simulink model "CDHRM_model_v1"  (R2019b)
settings: Solver=VariableStepAuto  StartTime=0.0  StopTime=10.0  RelTol=1e-3
InitFcn:
  | parameters.m
values from neighbouring files (symbols this model uses):
  a = 140/1000    (= 0.14)    [parameters.m]
  d = 23/2000    (= 0.0115)    [parameters.m]
  eta = 0.39    [parameters.m]
  g = 9.81    [parameters.m]
  J_L = 0.014 * 10e-7    (= 1.4e-08)    [parameters.m]
  J_R = 0.864 * 10e-7    (= 8.64e-07)    [parameters.m]
  k_m = 2560*100*pi/3    (= 268082.573106)    [parameters.m]
  k_trans = 0.36    [parameters.m]
  l_link = a-2*d    (= 0.117)    [parameters.m]
  m = 0.2    [parameters.m]
  mu_cable = 0.17    [parameters.m]
  n_0 = 9620*pi/30    (= 1007.40404425)    [parameters.m]
  p = 8/1000    (= 0.008)    [parameters.m]
  r = 20.5/1000    (= 0.0205)    [parameters.m]
  r_drum = 0.042    [parameters.m]
undefined symbols (not defined in the file or in its folder): d_drum
libraries: dspindex x18, dspinverses x1, simulink x1
(part 1 of 5)
settings Model: Creator=arund  LastModifiedBy=arund

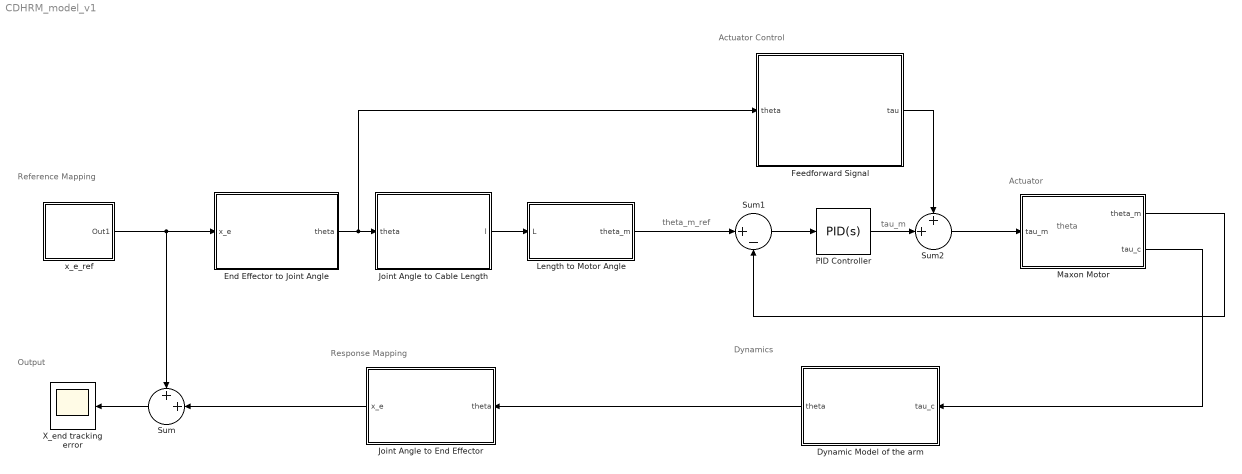
== system CDHRM_model_v1 ==
  note: Actuator
  note: theta_m_ref
  note: Dynamics
  note: Actuator Control
  note: Response Mapping
  note: Output
  note: Reference Mapping
  note: tau_m
  note: theta
  Dynamic Model of the arm : Subsystem
  End Effector to Joint Angle : Subsystem
  Feedforward Signal : Subsystem
  Joint Angle to Cable Length : Subsystem
  Joint Angle to End Effector : Subsystem
  Length to Motor Angle : Subsystem
  Maxon Motor : Subsystem
  PID Controller : simulink/Continuous/PID Controller  Controller=PID  Form=Parallel  TimeDomain=Continuous-time  SampleTime=-1  IntegratorMethod=Forward Euler  FilterMethod=Forward Euler  ControllerParametersSource=internal  P=74.7116129123462  I=0  D=0.141885827214998  UseFilter=on  N=364.6824066771  TunerSelectOption=Transfer Function Based (PID Tuner App)  InitialConditionSource=internal  InitialConditionForIntegrator=0  InitialConditionForFilter=0  DifferentiatorICPrevScaledInput=0  ExternalReset=none  TrackingMode=off  Kt=1  LimitOutput=off  UpperSaturationLimit=inf  LowerSaturationLimit=-inf  LinearizeAsGain=on  AntiWindupMode=none  Kb=1  POutMin=[]  POutMax=[]  IOutMin=[]  IOutMax=[]  DOutMin=[]  DOutMax=[]  NOutMin=[]  NOutMax=[]  SumOutMin=[]  SumOutMax=[]  SaturationOutMin=[]  SaturationOutMax=[]  PParamMin=[]  PParamMax=[]  IParamMin=[]  IParamMax=[]  DParamMin=[]  DParamMax=[]  NParamMin=[]  NParamMax=[]  KbParamMin=[]  KbParamMax=[]  KtParamMin=[]  KtParamMax=[]  KbOutMin=[]  KbOutMax=[]  KtOutMin=[]  KtOutMax=[]  IntegratorOutMin=[]  IntegratorOutMax=[]  FilterOutMin=[]  FilterOutMax=[]  SumI1OutMin=[]  SumI1OutMax=[]  SumI2OutMin=[]  SumI2OutMax=[]  SumI3OutMin=[]  SumI3OutMax=[]  SumI4OutMin=[]  SumI4OutMax=[]  SumDOutMin=[]  SumDOutMax=[]  DifferentiatorOutMin=[]  DifferentiatorOutMax=[]  FilterDiffOutCoefMin=[]  FilterDiffOutCoefMax=[]  ReciprocalOutMin=[]  ReciprocalOutMax=[]  SumDenOutMin=[]  SumDenOutMax=[]  SumNumOutMin=[]  SumNumOutMax=[]  DivideOutMin=[]  DivideOutMax=[]  IntegratorContinuousStateAttributes=''  IntegratorStateMustResolveToSignalObject=off  IntegratorRTWStateStorageClass=Auto  FilterContinuousStateAttributes=''  FilterStateMustResolveToSignalObject=off  FilterRTWStateStorageClass=Auto  ParallelPVariant=InternalParameters  IdealPVariant=Disabled  IVariant=InternalParameters  DVariant=InternalParameters  IntegratorVariant=Continuous  SatVariant=Disabled  AWVariant=Passthrough  PCopyVariant=Disabled  TRVariant=Disabled  FdbkBlocksVariant=Forward  IdealPFdbkVariant=Disabled  SatFdbkVariant=Disabled  DerivativeFilterVariant=ContFilter  NVariant=InternalParameters  NCopyVariant=Disabled  FilterICVariant=InternalICsFilter  IntegratorICVariant=InternalICs  ExternalResetVariant=Disabled  TRSumVariant=Passthrough  SumFdbkVariant=Disabled  SumVariant=Sum_PID
  Sum : Sum  Inputs=++|
  Sum1 : Sum  Inputs=|+-
  Sum2 : Sum  Inputs=++|
  X_end tracking error : Scope
  x_e_ref : Subsystem
  wires:
  Sum/1 -> X_end tracking error/1
  Joint Angle to End Effector/1(x_e) -> Sum/2
  Length to Motor Angle/1(theta_m) -> Sum1/1
  Sum1/1 -> PID Controller/1
  Maxon Motor/1(theta_m) -> Sum1/2
  Joint Angle to Cable Length/1(l) -> Length to Motor Angle/1(L)
  Sum2/1 -> Maxon Motor/1(tau_m)
  Dynamic Model of the arm/1(theta) -> Joint Angle to End Effector/1(theta)
  PID Controller/1 -> Sum2/2
  x_e_ref/1(Out1) -> End Effector to Joint Angle/1(x_e), Sum/1
  Maxon Motor/2(tau_c) -> Dynamic Model of the arm/1(tau_c)
  Feedforward Signal/1(tau) -> Sum2/1
  End Effector to Joint Angle/1(theta) -> Feedforward Signal/1(theta), Joint Angle to Cable Length/1(theta)

== system CDHRM_model_v1/Dynamic Model of the arm ==
  tau_c : Inport
  Integrator : Integrator
  Integrator1 : Integrator
  M_inv(theta) : Subsystem
  Matrix Multiply : Product  Multiplication=Matrix(*)
  h(theta,d_theta) : Subsystem
  theta : Outport
  wires:
  Integrator/1 -> h(theta,d_theta)/2(d_theta), Integrator1/1  "d_theta"
  Integrator1/1 -> h(theta,d_theta)/1(theta), M_inv(theta)/1(theta), theta/1
  Matrix Multiply/1 -> Integrator/1  "dd_theta"
  M_inv(theta)/1(M_inv) -> Matrix Multiply/1
  tau_c/1 -> M_inv(theta)/2(tau_c), h(theta,d_theta)/3(tau_c)
  h(theta,d_theta)/1(h) -> Matrix Multiply/2

== system CDHRM_model_v1/End Effector to Joint Angle ==
  x_e : Inport
  Constant1 : Constant  Value=a
  "End Effector to Joint Angle " : MATLAB Function  TreatAsAtomicUnit=on
  Memory : Memory
  Memory1 : Memory
  theta : Outport
  wires:
  "End Effector to Joint Angle "/1(theta) -> theta/1, Memory1/1
  Memory1/1 -> "End Effector to Joint Angle "/4(theta_prev)
  Memory/1 -> "End Effector to Joint Angle "/3(x_e_prev)
  x_e/1 -> Memory/1, "End Effector to Joint Angle "/2(x_e)
  Constant1/1 -> "End Effector to Joint Angle "/1(a)

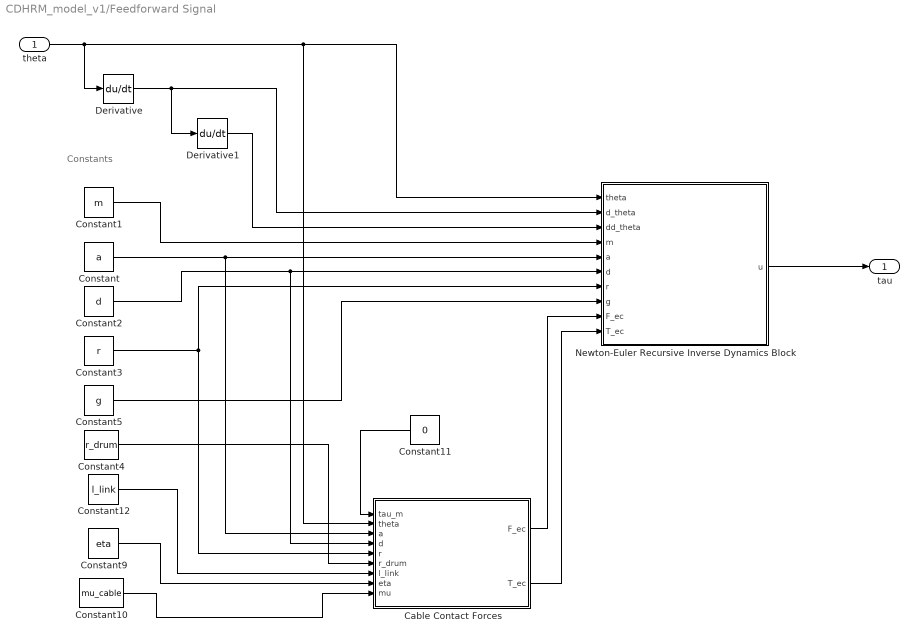
== system CDHRM_model_v1/Feedforward Signal ==
  note: Constants
  theta : Inport
  Cable Contact Forces : MATLAB Function  TreatAsAtomicUnit=on
  Constant : Constant  Value=a
  Constant1 : Constant  Value=m
  Constant10 : Constant  Value=mu_cable
  Constant11 : Constant  Value=0
  Constant12 : Constant  Value=l_link
  Constant2 : Constant  Value=d
  Constant3 : Constant  Value=r
  Constant4 : Constant  Value=r_drum
  Constant5 : Constant  Value=g
  Constant9 : Constant  Value=eta
  Derivative : Derivative  CoefficientInTFapproximation=0
  Derivative1 : Derivative  CoefficientInTFapproximation=0
  Newton-Euler Recursive Inverse Dynamics Block : MATLAB Function  TreatAsAtomicUnit=on
  tau : Outport
  wires:
  Constant/1 -> Cable Contact Forces/3(a), Newton-Euler Recursive Inverse Dynamics Block/5(a)
  Constant9/1 -> Cable Contact Forces/8(eta)
  Constant4/1 -> Cable Contact Forces/6(r_drum)
  theta/1 -> Derivative/1, Cable Contact Forces/2(theta), Newton-Euler Recursive Inverse Dynamics Block/1(theta)
  Constant2/1 -> Cable Contact Forces/4(d), Newton-Euler Recursive Inverse Dynamics Block/6(d)
  Constant3/1 -> Cable Contact Forces/5(r), Newton-Euler Recursive Inverse Dynamics Block/7(r)
  Constant10/1 -> Cable Contact Forces/9(mu)
  Constant1/1 -> Newton-Euler Recursive Inverse Dynamics Block/4(m)
  Constant5/1 -> Newton-Euler Recursive Inverse Dynamics Block/8(g)
  Newton-Euler Recursive Inverse Dynamics Block/1(u) -> tau/1
  Cable Contact Forces/2(T_ec) -> Newton-Euler Recursive Inverse Dynamics Block/10(T_ec)
  Cable Contact Forces/1(F_ec) -> Newton-Euler Recursive Inverse Dynamics Block/9(F_ec)
  Constant12/1 -> Cable Contact Forces/7(l_link)
  Constant11/1 -> Cable Contact Forces/1(tau_m)
  Derivative/1 -> Derivative1/1, Newton-Euler Recursive Inverse Dynamics Block/2(d_theta)
  Derivative1/1 -> Newton-Euler Recursive Inverse Dynamics Block/3(dd_theta)

== system CDHRM_model_v1/Joint Angle to Cable Length ==
  theta : Inport
  Joint Angle to Cable Length : MATLAB Function  TreatAsAtomicUnit=on
  theta to phi : MATLAB Function  TreatAsAtomicUnit=on
  l : Outport
  wires:
  Joint Angle to Cable Length/1(l) -> l/1
  theta/1 -> theta to phi/1(theta)
  theta to phi/1(phi_p) -> Joint Angle to Cable Length/1(phi_p)
  theta to phi/2(phi_d) -> Joint Angle to Cable Length/2(phi_d)

== system CDHRM_model_v1/Joint Angle to End Effector ==
  theta : Inport
  Constant1 : Constant  Value=a
  Derivative : Derivative  CoefficientInTFapproximation=0
  Integrator : Integrator
  "Jacobian of theta " : MATLAB Function  TreatAsAtomicUnit=on
  MatrixMultiply : Product  Multiplication=Matrix(*)
  x_e : Outport
  wires:
  Derivative/1 -> MatrixMultiply/2
  "Jacobian of theta "/1(J) -> MatrixMultiply/1
  Constant1/1 -> "Jacobian of theta "/1(a)
  theta/1 -> "Jacobian of theta "/2(theta), Derivative/1
  MatrixMultiply/1 -> Integrator/1
  Integrator/1 -> x_e/1

== system CDHRM_model_v1/Length to Motor Angle ==
  L : Inport
  Constant : Constant  Value=p
  Constant2 : Constant  Value=d_drum
  Divide : Product  Inputs=*/
  Transmission ratio : Subsystem
  theta_m : Outport
  wires:
  L/1 -> Divide/1
  Constant2/1 -> Transmission ratio/2(d_drum)
  Constant/1 -> Transmission ratio/1(p)
  Transmission ratio/1(k) -> Divide/2
  Divide/1 -> theta_m/1

== system CDHRM_model_v1/Maxon Motor ==
  tau_m : Inport
  Motor : Subsystem
  Speed to Torque : Subsystem
  theta_m : Outport
  tau_c : Outport  Port=2
  wires:
  tau_m/1 -> Motor/1(tau_m)
  Motor/1(Out1) -> theta_m/1
  Motor/2(Out2) -> Speed to Torque/1(d_theta_m)
  Speed to Torque/1(tau_c) -> tau_c/1

== system CDHRM_model_v1/x_e_ref ==
  Mux : Mux  Inputs=6
  X_end_ref{,1..4} (5 alike) : Step  After=0  SampleTime=0
  X_end_ref5 : Step  After=0.1  SampleTime=0
  Out1 : Outport
  wires:
  Mux/1 -> Out1/1
  X_end_ref5/1 -> Mux/1
  X_end_ref/1 -> Mux/2
  X_end_ref1/1 -> Mux/3
  X_end_ref2/1 -> Mux/4
  X_end_ref3/1 -> Mux/5
  X_end_ref4/1 -> Mux/6

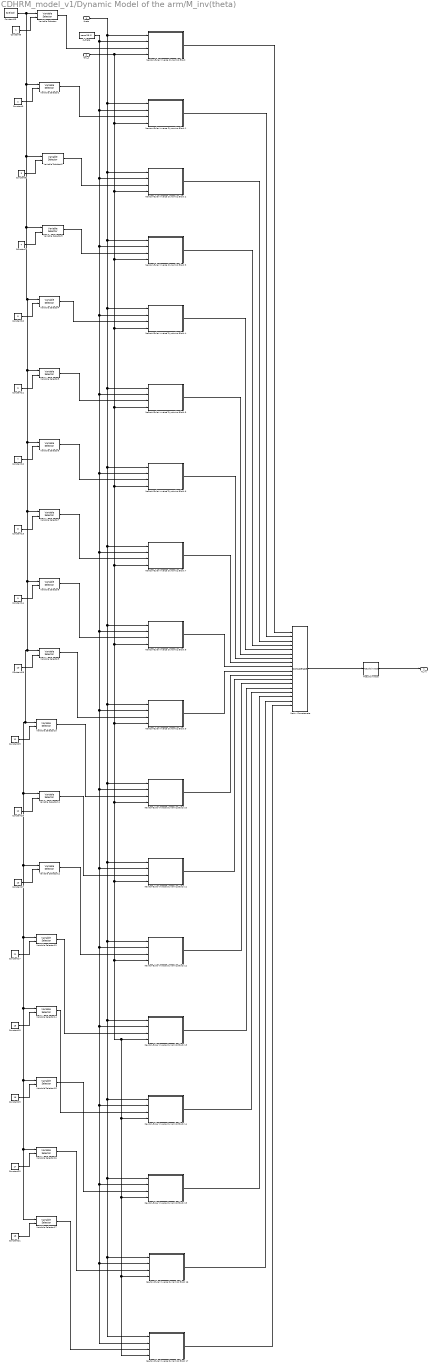
== system CDHRM_model_v1/Dynamic Model of the arm/M_inv(theta) ==
  theta : Inport
  tau_c : Inport  Port=2
  Constant10 : Constant  Value=5
  Constant11 : Constant  Value=6
  Constant12 : Constant  Value=7
  Constant13 : Constant  Value=8
  Constant14 : Constant  Value=9
  Constant15 : Constant  Value=eye(18)
  Constant17 : Constant  Value=14
  Constant18 : Constant  Value=15
  Constant19 : Constant  Value=16
  Constant20 : Constant  Value=17
  Constant21 : Constant  Value=18
  Constant26 : Constant  Value=12
  Constant27 : Constant  Value=13
  Constant28 : Constant  Value=10
  Constant29 : Constant  Value=11
  Constant6 : Constant  Value=3
  Constant7 : Constant  Value=4
  Constant8 : Constant
  Constant9 : Constant  Value=2
  Matrix Concatenate : Concatenate  NumInputs=18  Mode=Multidimensional array  ConcatenateDimension=2
  "Newton-Euler Inverse Dynamics Block " : Subsystem
  Newton-Euler Inverse Dynamics Block 1 : Subsystem
  Newton-Euler Inverse Dynamics Block 10 : Subsystem
  Newton-Euler Inverse Dynamics Block 11 : Subsystem
  Newton-Euler Inverse Dynamics Block 12 : Subsystem
  Newton-Euler Inverse Dynamics Block 13 : Subsystem
  Newton-Euler Inverse Dynamics Block 14 : Subsystem
  Newton-Euler Inverse Dynamics Block 15 : Subsystem
  Newton-Euler Inverse Dynamics Block 16 : Subsystem
  Newton-Euler Inverse Dynamics Block 17 : Subsystem
  Newton-Euler Inverse Dynamics Block 2 : Subsystem
  Newton-Euler Inverse Dynamics Block 3 : Subsystem
  Newton-Euler Inverse Dynamics Block 4 : Subsystem
  Newton-Euler Inverse Dynamics Block 5 : Subsystem
  Newton-Euler Inverse Dynamics Block 6 : Subsystem
  Newton-Euler Inverse Dynamics Block 7 : Subsystem
  Newton-Euler Inverse Dynamics Block 8 : Subsystem
  Newton-Euler Inverse Dynamics Block 9 : Subsystem
  Pseudoinverse : dspinverses/Pseudoinverse  wanterr=off  SimulateUsing=Interpreted execution
      settings: SourceProductName=DSP System Toolbox  SourceProductBaseCode=DS
  Variable Selector{,1..17} (18 alike) : dspindex/Variable Selector  NumInputs=1  rowsOrCols=Columns  IdxMode=Variable  Elements=[1 3]  ZerOneIdxMode=One-based  errmode=Clip Index  FillMode=on  FillValues=0
  d_theta : Constant  Value=zeros(18,1)
  M_inv : Outport
  wires:
  Variable Selector/1 -> "Newton-Euler Inverse Dynamics Block "/3(dd_theta)
  Constant8/1 -> Variable Selector/2
  Variable Selector1/1 -> Newton-Euler Inverse Dynamics Block 1/3(dd_theta)
  Constant9/1 -> Variable Selector1/2
  Matrix Concatenate/1 -> Pseudoinverse/1
  Constant6/1 -> Variable Selector2/2
  Variable Selector2/1 -> Newton-Euler Inverse Dynamics Block 2/3(dd_theta)
  Constant7/1 -> Variable Selector3/2
  Variable Selector3/1 -> Newton-Euler Inverse Dynamics Block 3/3(dd_theta)
  Constant10/1 -> Variable Selector4/2
  Variable Selector4/1 -> Newton-Euler Inverse Dynamics Block 4/3(dd_theta)
  Constant11/1 -> Variable Selector5/2
  Variable Selector5/1 -> Newton-Euler Inverse Dynamics Block 5/3(dd_theta)
  Constant12/1 -> Variable Selector6/2
  Variable Selector6/1 -> Newton-Euler Inverse Dynamics Block 6/3(dd_theta)
  Constant13/1 -> Variable Selector7/2
  Variable Selector7/1 -> Newton-Euler Inverse Dynamics Block 7/3(dd_theta)
  Constant14/1 -> Variable Selector8/2
  Variable Selector8/1 -> Newton-Euler Inverse Dynamics Block 8/3(dd_theta)
  Pseudoinverse/1 -> M_inv/1
  Variable Selector11/1 -> Newton-Euler Inverse Dynamics Block 11/3(dd_theta)
  Constant26/1 -> Variable Selector11/2
  Variable Selector14/1 -> Newton-Euler Inverse Dynamics Block 14/3(dd_theta)
  Constant18/1 -> Variable Selector14/2
  Variable Selector17/1 -> Newton-Euler Inverse Dynamics Block 17/3(dd_theta)
  Constant21/1 -> Variable Selector17/2
  Constant15/1 -> Variable Selector9/1, Variable Selector10/1, Variable Selector17/1, Variable Selector16/1, Variable Selector15/1, Variable Selector14/1, Variable Selector13/1, Variable Selector12/1, Variable Selector11/1, Variable Selector8/1, Variable Selector7/1, Variable Selector6/1, Variable Selector5/1, Variable Selector4/1, Variable Selector3/1, Variable Selector2/1, Variable Selector1/1, Variable Selector/1
  d_theta/1 -> "Newton-Euler Inverse Dynamics Block "/2(d_theta), Newton-Euler Inverse Dynamics Block 6/2(d_theta), Newton-Euler Inverse Dynamics Block 7/2(d_theta), Newton-Euler Inverse Dynamics Block 8/2(d_theta), Newton-Euler Inverse Dynamics Block 9/2(d_theta), Newton-Euler Inverse Dynamics Block 11/2(d_theta), Newton-Euler Inverse Dynamics Block 12/2(d_theta), Newton-Euler Inverse Dynamics Block 17/2(d_theta), Newton-Euler Inverse Dynamics Block 16/2(d_theta), Newton-Euler Inverse Dynamics Block 15/2(d_theta), Newton-Euler Inverse Dynamics Block 14/2(d_theta), Newton-Euler Inverse Dynamics Block 13/2(d_theta), Newton-Euler Inverse Dynamics Block 10/2(d_theta), Newton-Euler Inverse Dynamics Block 5/2(d_theta), Newton-Euler Inverse Dynamics Block 4/2(d_theta), Newton-Euler Inverse Dynamics Block 3/2(d_theta), Newton-Euler Inverse Dynamics Block 2/2(d_theta), Newton-Euler Inverse Dynamics Block 1/2(d_theta)
  theta/1 -> "Newton-Euler Inverse Dynamics Block "/1(theta), Newton-Euler Inverse Dynamics Block 1/1(theta), Newton-Euler Inverse Dynamics Block 3/1(theta), Newton-Euler Inverse Dynamics Block 4/1(theta), Newton-Euler Inverse Dynamics Block 5/1(theta), Newton-Euler Inverse Dynamics Block 6/1(theta), Newton-Euler Inverse Dynamics Block 7/1(theta), Newton-Euler Inverse Dynamics Block 8/1(theta), Newton-Euler Inverse Dynamics Block 9/1(theta), Newton-Euler Inverse Dynamics Block 10/1(theta), Newton-Euler Inverse Dynamics Block 11/1(theta), Newton-Euler Inverse Dynamics Block 12/1(theta), Newton-Euler Inverse Dynamics Block 13/1(theta), Newton-Euler Inverse Dynamics Block 14/1(theta), Newton-Euler Inverse Dynamics Block 16/1(theta), Newton-Euler Inverse Dynamics Block 17/1(theta), Newton-Euler Inverse Dynamics Block 15/1(theta), Newton-Euler Inverse Dynamics Block 2/1(theta)
  Constant28/1 -> Variable Selector9/2
  Variable Selector13/1 -> Newton-Euler Inverse Dynamics Block 13/3(dd_theta)
  Constant17/1 -> Variable Selector13/2
  Constant20/1 -> Variable Selector16/2
  Constant19/1 -> Variable Selector15/2
  Constant29/1 -> Variable Selector10/2
  Variable Selector10/1 -> Newton-Euler Inverse Dynamics Block 10/3(dd_theta)
  Variable Selector9/1 -> Newton-Euler Inverse Dynamics Block 9/3(dd_theta)
  Constant27/1 -> Variable Selector12/2
  Variable Selector12/1 -> Newton-Euler Inverse Dynamics Block 12/3(dd_theta)
  Variable Selector15/1 -> Newton-Euler Inverse Dynamics Block 15/3(dd_theta)
  Variable Selector16/1 -> Newton-Euler Inverse Dynamics Block 16/3(dd_theta)
  tau_c/1 -> Newton-Euler Inverse Dynamics Block 6/4(tau_c), Newton-Euler Inverse Dynamics Block 11/4(tau_c), Newton-Euler Inverse Dynamics Block 12/4(tau_c), Newton-Euler Inverse Dynamics Block 13/4(tau_c), Newton-Euler Inverse Dynamics Block 14/4(tau_c), Newton-Euler Inverse Dynamics Block 15/4(tau_c), Newton-Euler Inverse Dynamics Block 17/4(tau_c), Newton-Euler Inverse Dynamics Block 16/4(tau_c), Newton-Euler Inverse Dynamics Block 10/4(tau_c), Newton-Euler Inverse Dynamics Block 9/4(tau_c), Newton-Euler Inverse Dynamics Block 8/4(tau_c), Newton-Euler Inverse Dynamics Block 7/4(tau_c), Newton-Euler Inverse Dynamics Block 5/4(tau_c), Newton-Euler Inverse Dynamics Block 4/4(tau_c), Newton-Euler Inverse Dynamics Block 3/4(tau_c), Newton-Euler Inverse Dynamics Block 2/4(tau_c), Newton-Euler Inverse Dynamics Block 1/4(tau_c), "Newton-Euler Inverse Dynamics Block "/4(tau_c)
  "Newton-Euler Inverse Dynamics Block "/1(tau) -> Matrix Concatenate/1
  Newton-Euler Inverse Dynamics Block 1/1(tau) -> Matrix Concatenate/2
  Newton-Euler Inverse Dynamics Block 2/1(tau) -> Matrix Concatenate/3
  Newton-Euler Inverse Dynamics Block 3/1(tau) -> Matrix Concatenate/4
  Newton-Euler Inverse Dynamics Block 4/1(tau) -> Matrix Concatenate/5
  Newton-Euler Inverse Dynamics Block 5/1(tau) -> Matrix Concatenate/6
  Newton-Euler Inverse Dynamics Block 6/1(tau) -> Matrix Concatenate/7
  Newton-Euler Inverse Dynamics Block 7/1(tau) -> Matrix Concatenate/8
  Newton-Euler Inverse Dynamics Block 8/1(tau) -> Matrix Concatenate/9
  Newton-Euler Inverse Dynamics Block 9/1(tau) -> Matrix Concatenate/10
  Newton-Euler Inverse Dynamics Block 10/1(tau) -> Matrix Concatenate/11
  Newton-Euler Inverse Dynamics Block 11/1(tau) -> Matrix Concatenate/12
  Newton-Euler Inverse Dynamics Block 12/1(tau) -> Matrix Concatenate/13
  Newton-Euler Inverse Dynamics Block 13/1(tau) -> Matrix Concatenate/14
  Newton-Euler Inverse Dynamics Block 14/1(tau) -> Matrix Concatenate/15
  Newton-Euler Inverse Dynamics Block 15/1(tau) -> Matrix Concatenate/16
  Newton-Euler Inverse Dynamics Block 16/1(tau) -> Matrix Concatenate/17
  Newton-Euler Inverse Dynamics Block 17/1(tau) -> Matrix Concatenate/18

== system CDHRM_model_v1/Dynamic Model of the arm/h(theta,d_theta) ==
  theta : Inport
  d_theta : Inport  Port=2
  tau_c : Inport  Port=3
  "Newton-Euler Inverse Dynamics Block " : Subsystem
  dd_theta : Constant  Value=zeros(18,1)
  h : Outport
  wires:
  "Newton-Euler Inverse Dynamics Block "/1(tau) -> h/1
  dd_theta/1 -> "Newton-Euler Inverse Dynamics Block "/3(dd_theta)
  d_theta/1 -> "Newton-Euler Inverse Dynamics Block "/2(d_theta)
  theta/1 -> "Newton-Euler Inverse Dynamics Block "/1(theta)
  tau_c/1 -> "Newton-Euler Inverse Dynamics Block "/4(tau_c)

== system CDHRM_model_v1/Length to Motor Angle/Transmission ratio ==
  p : Inport
  d_drum : Inport  Port=2
  Multiply : Gain  Gain=k_trans
  Square : Math  Operator=square  SignedPower=off  SaturateOnIntegerOverflow=on
  Square Root : Sqrt  SaturateOnIntegerOverflow=on
  Square1 : Math  Operator=square  SignedPower=off  SaturateOnIntegerOverflow=on
  Sum : Sum
  k : Outport
  wires:
  Square/1 -> Sum/1
  p/1 -> Square/1
  d_drum/1 -> Square1/1
  Square1/1 -> Sum/2
  Sum/1 -> Square Root/1
  Square Root/1 -> Multiply/1
  Multiply/1 -> k/1

== system CDHRM_model_v1/Maxon Motor/Motor ==
  tau_m : Inport
  Add : Sum
  Constant1 : Constant  Value=J_L
  Constant2 : Constant  Value=J_R
  Integrator : Integrator
  Integrator1 : Integrator
  Product : Product  Inputs=*/
  Out1 : Outport
  Out2 : Outport  Port=2
  wires:
  Integrator/1 -> Out1/1
  Integrator1/1 -> Out2/1, Integrator/1
  Product/1 -> Integrator1/1
  Constant2/1 -> Add/2
  tau_m/1 -> Product/1
  Add/1 -> Product/2
  Constant1/1 -> Add/1

== system CDHRM_model_v1/Maxon Motor/Speed to Torque ==
  d_theta_m : Inport
  Constant : Constant  Value=k_m
  Constant1 : Constant  Value=n_0
  Divide : Product  Inputs=*/
  Subtract : Sum  Inputs=+-
  tau_c : Outport
  wires:
  Constant/1 -> Divide/2
  Constant1/1 -> Subtract/1
  Divide/1 -> tau_c/1
  Subtract/1 -> Divide/1
  d_theta_m/1 -> Subtract/2

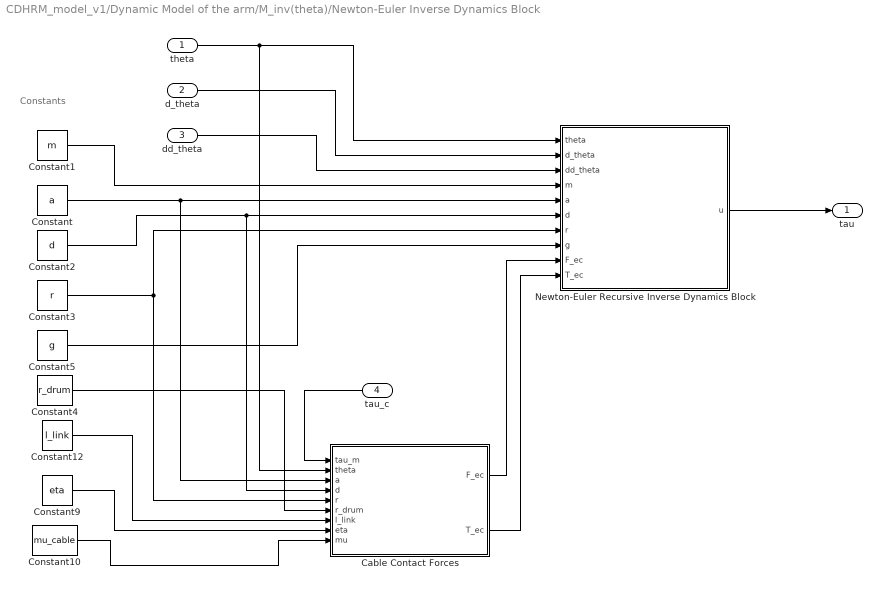
== system CDHRM_model_v1/Dynamic Model of the arm/M_inv(theta)/Newton-Euler Inverse Dynamics Block  ==
  note: Constants
  theta : Inport
  d_theta : Inport  Port=2
  dd_theta : Inport  Port=3
  tau_c : Inport  Port=4
  Cable Contact Forces : MATLAB Function  TreatAsAtomicUnit=on
  Constant : Constant  Value=a
  Constant1 : Constant  Value=m
  Constant10 : Constant  Value=mu_cable
  Constant12 : Constant  Value=l_link
  Constant2 : Constant  Value=d
  Constant3 : Constant  Value=r
  Constant4 : Constant  Value=r_drum
  Constant5 : Constant  Value=g
  Constant9 : Constant  Value=eta
  Newton-Euler Recursive Inverse Dynamics Block : MATLAB Function  TreatAsAtomicUnit=on
  tau : Outport
  wires:
  Constant/1 -> Cable Contact Forces/3(a), Newton-Euler Recursive Inverse Dynamics Block/5(a)
  dd_theta/1 -> Newton-Euler Recursive Inverse Dynamics Block/3(dd_theta)
  Constant9/1 -> Cable Contact Forces/8(eta)
  Constant4/1 -> Cable Contact Forces/6(r_drum)
  theta/1 -> Newton-Euler Recursive Inverse Dynamics Block/1(theta), Cable Contact Forces/2(theta)
  Constant2/1 -> Cable Contact Forces/4(d), Newton-Euler Recursive Inverse Dynamics Block/6(d)
  Constant3/1 -> Cable Contact Forces/5(r), Newton-Euler Recursive Inverse Dynamics Block/7(r)
  Constant10/1 -> Cable Contact Forces/9(mu)
  d_theta/1 -> Newton-Euler Recursive Inverse Dynamics Block/2(d_theta)
  Constant1/1 -> Newton-Euler Recursive Inverse Dynamics Block/4(m)
  Constant5/1 -> Newton-Euler Recursive Inverse Dynamics Block/8(g)
  Newton-Euler Recursive Inverse Dynamics Block/1(u) -> tau/1
  Cable Contact Forces/2(T_ec) -> Newton-Euler Recursive Inverse Dynamics Block/10(T_ec)
  Cable Contact Forces/1(F_ec) -> Newton-Euler Recursive Inverse Dynamics Block/9(F_ec)
  Constant12/1 -> Cable Contact Forces/7(l_link)
  tau_c/1 -> Cable Contact Forces/1(tau_m)

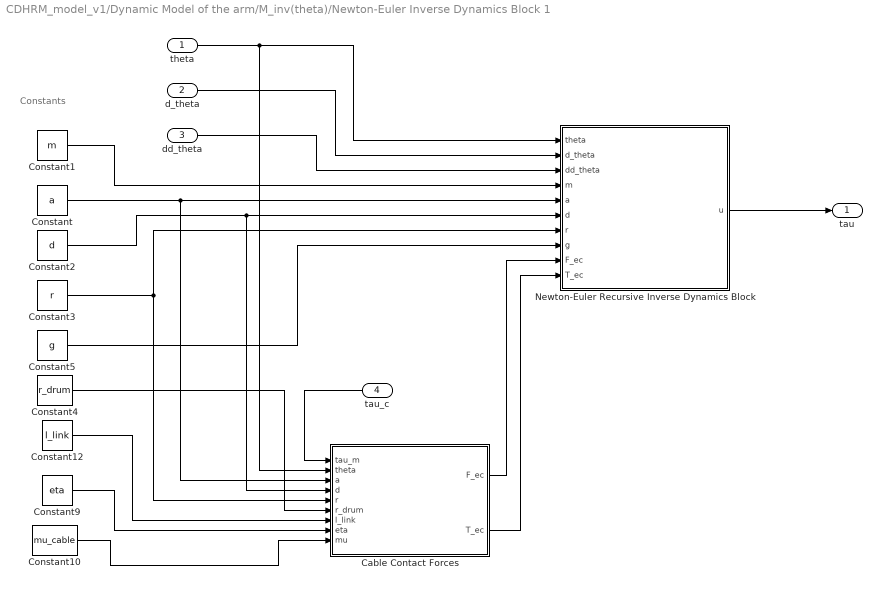
== system CDHRM_model_v1/Dynamic Model of the arm/M_inv(theta)/Newton-Euler Inverse Dynamics Block 1 ==
  note: Constants
  theta : Inport
  d_theta : Inport  Port=2
  dd_theta : Inport  Port=3
  tau_c : Inport  Port=4
  Cable Contact Forces : MATLAB Function  TreatAsAtomicUnit=on
  Constant : Constant  Value=a
  Constant1 : Constant  Value=m
  Constant10 : Constant  Value=mu_cable
  Constant12 : Constant  Value=l_link
  Constant2 : Constant  Value=d
  Constant3 : Constant  Value=r
  Constant4 : Constant  Value=r_drum
  Constant5 : Constant  Value=g
  Constant9 : Constant  Value=eta
  Newton-Euler Recursive Inverse Dynamics Block : MATLAB Function  TreatAsAtomicUnit=on
  tau : Outport
  wires:
  Constant/1 -> Cable Contact Forces/3(a), Newton-Euler Recursive Inverse Dynamics Block/5(a)
  dd_theta/1 -> Newton-Euler Recursive Inverse Dynamics Block/3(dd_theta)
  Constant9/1 -> Cable Contact Forces/8(eta)
  Constant4/1 -> Cable Contact Forces/6(r_drum)
  theta/1 -> Newton-Euler Recursive Inverse Dynamics Block/1(theta), Cable Contact Forces/2(theta)
  Constant2/1 -> Cable Contact Forces/4(d), Newton-Euler Recursive Inverse Dynamics Block/6(d)
  Constant3/1 -> Cable Contact Forces/5(r), Newton-Euler Recursive Inverse Dynamics Block/7(r)
  Constant10/1 -> Cable Contact Forces/9(mu)
  d_theta/1 -> Newton-Euler Recursive Inverse Dynamics Block/2(d_theta)
  Constant1/1 -> Newton-Euler Recursive Inverse Dynamics Block/4(m)
  Constant5/1 -> Newton-Euler Recursive Inverse Dynamics Block/8(g)
  Newton-Euler Recursive Inverse Dynamics Block/1(u) -> tau/1
  Cable Contact Forces/2(T_ec) -> Newton-Euler Recursive Inverse Dynamics Block/10(T_ec)
  Cable Contact Forces/1(F_ec) -> Newton-Euler Recursive Inverse Dynamics Block/9(F_ec)
  Constant12/1 -> Cable Contact Forces/7(l_link)
  tau_c/1 -> Cable Contact Forces/1(tau_m)

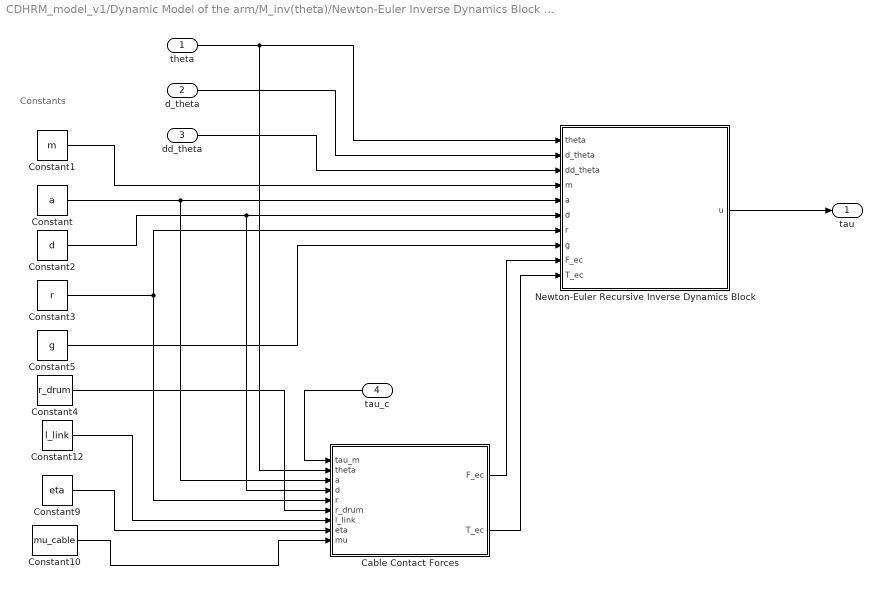
== system CDHRM_model_v1/Dynamic Model of the arm/M_inv(theta)/Newton-Euler Inverse Dynamics Block 10 ==
  note: Constants
  theta : Inport
  d_theta : Inport  Port=2
  dd_theta : Inport  Port=3
  tau_c : Inport  Port=4
  Cable Contact Forces : MATLAB Function  TreatAsAtomicUnit=on
  Constant : Constant  Value=a
  Constant1 : Constant  Value=m
  Constant10 : Constant  Value=mu_cable
  Constant12 : Constant  Value=l_link
  Constant2 : Constant  Value=d
  Constant3 : Constant  Value=r
  Constant4 : Constant  Value=r_drum
  Constant5 : Constant  Value=g
  Constant9 : Constant  Value=eta
  Newton-Euler Recursive Inverse Dynamics Block : MATLAB Function  TreatAsAtomicUnit=on
  tau : Outport
  wires:
  Constant/1 -> Cable Contact Forces/3(a), Newton-Euler Recursive Inverse Dynamics Block/5(a)
  dd_theta/1 -> Newton-Euler Recursive Inverse Dynamics Block/3(dd_theta)
  Constant9/1 -> Cable Contact Forces/8(eta)
  Constant4/1 -> Cable Contact Forces/6(r_drum)
  theta/1 -> Newton-Euler Recursive Inverse Dynamics Block/1(theta), Cable Contact Forces/2(theta)
  Constant2/1 -> Cable Contact Forces/4(d), Newton-Euler Recursive Inverse Dynamics Block/6(d)
  Constant3/1 -> Cable Contact Forces/5(r), Newton-Euler Recursive Inverse Dynamics Block/7(r)
  Constant10/1 -> Cable Contact Forces/9(mu)
  d_theta/1 -> Newton-Euler Recursive Inverse Dynamics Block/2(d_theta)
  Constant1/1 -> Newton-Euler Recursive Inverse Dynamics Block/4(m)
  Constant5/1 -> Newton-Euler Recursive Inverse Dynamics Block/8(g)
  Newton-Euler Recursive Inverse Dynamics Block/1(u) -> tau/1
  Cable Contact Forces/2(T_ec) -> Newton-Euler Recursive Inverse Dynamics Block/10(T_ec)
  Cable Contact Forces/1(F_ec) -> Newton-Euler Recursive Inverse Dynamics Block/9(F_ec)
  Constant12/1 -> Cable Contact Forces/7(l_link)
  tau_c/1 -> Cable Contact Forces/1(tau_m)

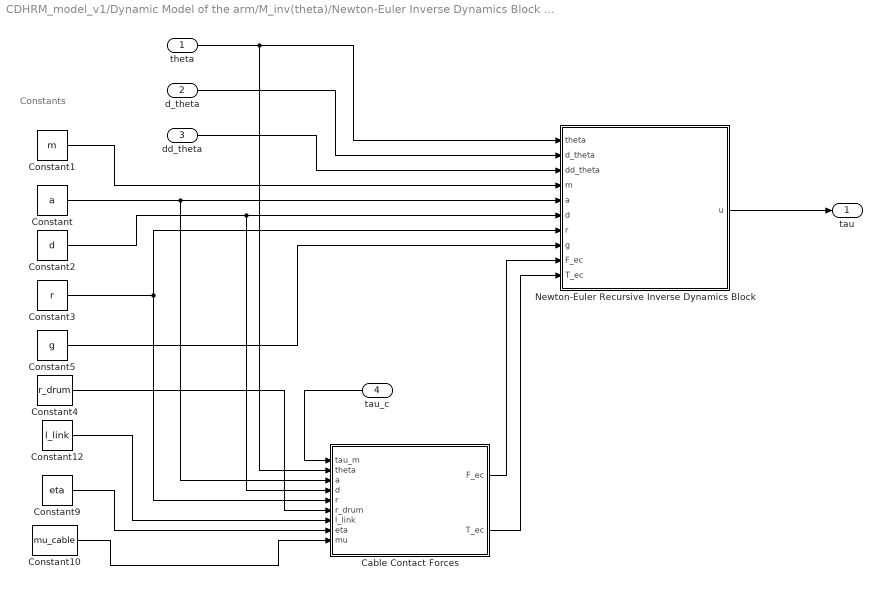
== system CDHRM_model_v1/Dynamic Model of the arm/M_inv(theta)/Newton-Euler Inverse Dynamics Block 11 ==
  note: Constants
  theta : Inport
  d_theta : Inport  Port=2
  dd_theta : Inport  Port=3
  tau_c : Inport  Port=4
  Cable Contact Forces : MATLAB Function  TreatAsAtomicUnit=on
  Constant : Constant  Value=a
  Constant1 : Constant  Value=m
  Constant10 : Constant  Value=mu_cable
  Constant12 : Constant  Value=l_link
  Constant2 : Constant  Value=d
  Constant3 : Constant  Value=r
  Constant4 : Constant  Value=r_drum
  Constant5 : Constant  Value=g
  Constant9 : Constant  Value=eta
  Newton-Euler Recursive Inverse Dynamics Block : MATLAB Function  TreatAsAtomicUnit=on
  tau : Outport
  wires:
  Constant/1 -> Cable Contact Forces/3(a), Newton-Euler Recursive Inverse Dynamics Block/5(a)
  dd_theta/1 -> Newton-Euler Recursive Inverse Dynamics Block/3(dd_theta)
  Constant9/1 -> Cable Contact Forces/8(eta)
  Constant4/1 -> Cable Contact Forces/6(r_drum)
  theta/1 -> Newton-Euler Recursive Inverse Dynamics Block/1(theta), Cable Contact Forces/2(theta)
  Constant2/1 -> Cable Contact Forces/4(d), Newton-Euler Recursive Inverse Dynamics Block/6(d)
  Constant3/1 -> Cable Contact Forces/5(r), Newton-Euler Recursive Inverse Dynamics Block/7(r)
  Constant10/1 -> Cable Contact Forces/9(mu)
  d_theta/1 -> Newton-Euler Recursive Inverse Dynamics Block/2(d_theta)
  Constant1/1 -> Newton-Euler Recursive Inverse Dynamics Block/4(m)
  Constant5/1 -> Newton-Euler Recursive Inverse Dynamics Block/8(g)
  Newton-Euler Recursive Inverse Dynamics Block/1(u) -> tau/1
  Cable Contact Forces/2(T_ec) -> Newton-Euler Recursive Inverse Dynamics Block/10(T_ec)
  Cable Contact Forces/1(F_ec) -> Newton-Euler Recursive Inverse Dynamics Block/9(F_ec)
  Constant12/1 -> Cable Contact Forces/7(l_link)
  tau_c/1 -> Cable Contact Forces/1(tau_m)

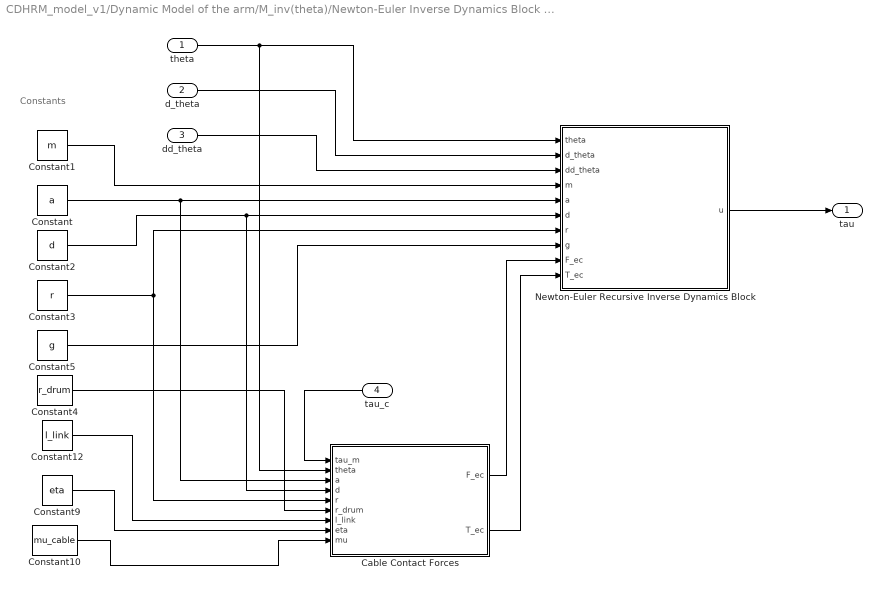
== system CDHRM_model_v1/Dynamic Model of the arm/M_inv(theta)/Newton-Euler Inverse Dynamics Block 12 ==
  note: Constants
  theta : Inport
  d_theta : Inport  Port=2
  dd_theta : Inport  Port=3
  tau_c : Inport  Port=4
  Cable Contact Forces : MATLAB Function  TreatAsAtomicUnit=on
  Constant : Constant  Value=a
  Constant1 : Constant  Value=m
  Constant10 : Constant  Value=mu_cable
  Constant12 : Constant  Value=l_link
  Constant2 : Constant  Value=d
  Constant3 : Constant  Value=r
  Constant4 : Constant  Value=r_drum
  Constant5 : Constant  Value=g
  Constant9 : Constant  Value=eta
  Newton-Euler Recursive Inverse Dynamics Block : MATLAB Function  TreatAsAtomicUnit=on
  tau : Outport
  wires:
  Constant/1 -> Cable Contact Forces/3(a), Newton-Euler Recursive Inverse Dynamics Block/5(a)
  dd_theta/1 -> Newton-Euler Recursive Inverse Dynamics Block/3(dd_theta)
  Constant9/1 -> Cable Contact Forces/8(eta)
  Constant4/1 -> Cable Contact Forces/6(r_drum)
  theta/1 -> Newton-Euler Recursive Inverse Dynamics Block/1(theta), Cable Contact Forces/2(theta)
  Constant2/1 -> Cable Contact Forces/4(d), Newton-Euler Recursive Inverse Dynamics Block/6(d)
  Constant3/1 -> Cable Contact Forces/5(r), Newton-Euler Recursive Inverse Dynamics Block/7(r)
  Constant10/1 -> Cable Contact Forces/9(mu)
  d_theta/1 -> Newton-Euler Recursive Inverse Dynamics Block/2(d_theta)
  Constant1/1 -> Newton-Euler Recursive Inverse Dynamics Block/4(m)
  Constant5/1 -> Newton-Euler Recursive Inverse Dynamics Block/8(g)
  Newton-Euler Recursive Inverse Dynamics Block/1(u) -> tau/1
  Cable Contact Forces/2(T_ec) -> Newton-Euler Recursive Inverse Dynamics Block/10(T_ec)
  Cable Contact Forces/1(F_ec) -> Newton-Euler Recursive Inverse Dynamics Block/9(F_ec)
  Constant12/1 -> Cable Contact Forces/7(l_link)
  tau_c/1 -> Cable Contact Forces/1(tau_m)

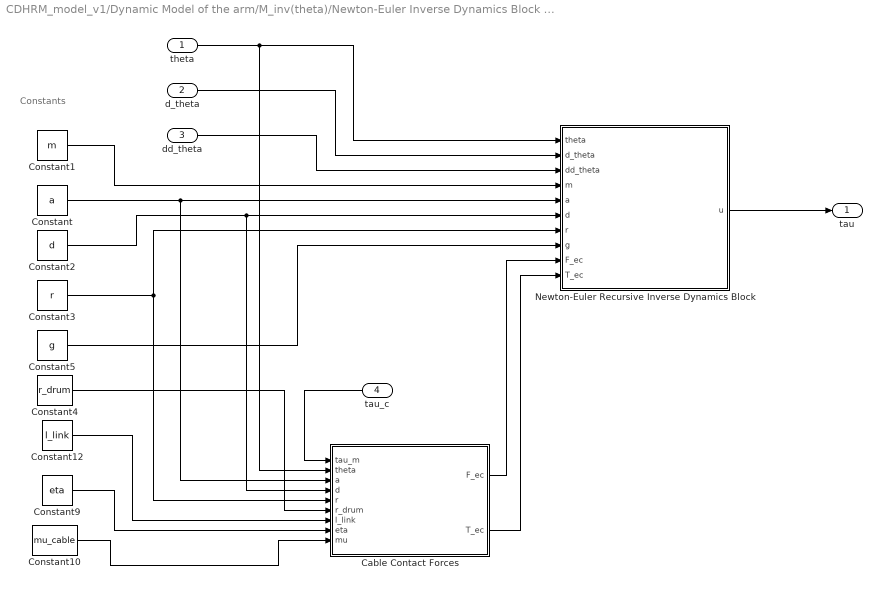
== system CDHRM_model_v1/Dynamic Model of the arm/M_inv(theta)/Newton-Euler Inverse Dynamics Block 13 ==
  note: Constants
  theta : Inport
  d_theta : Inport  Port=2
  dd_theta : Inport  Port=3
  tau_c : Inport  Port=4
  Cable Contact Forces : MATLAB Function  TreatAsAtomicUnit=on
  Constant : Constant  Value=a
  Constant1 : Constant  Value=m
  Constant10 : Constant  Value=mu_cable
  Constant12 : Constant  Value=l_link
  Constant2 : Constant  Value=d
  Constant3 : Constant  Value=r
  Constant4 : Constant  Value=r_drum
  Constant5 : Constant  Value=g
  Constant9 : Constant  Value=eta
  Newton-Euler Recursive Inverse Dynamics Block : MATLAB Function  TreatAsAtomicUnit=on
  tau : Outport
  wires:
  Constant/1 -> Cable Contact Forces/3(a), Newton-Euler Recursive Inverse Dynamics Block/5(a)
  dd_theta/1 -> Newton-Euler Recursive Inverse Dynamics Block/3(dd_theta)
  Constant9/1 -> Cable Contact Forces/8(eta)
  Constant4/1 -> Cable Contact Forces/6(r_drum)
  theta/1 -> Newton-Euler Recursive Inverse Dynamics Block/1(theta), Cable Contact Forces/2(theta)
  Constant2/1 -> Cable Contact Forces/4(d), Newton-Euler Recursive Inverse Dynamics Block/6(d)
  Constant3/1 -> Cable Contact Forces/5(r), Newton-Euler Recursive Inverse Dynamics Block/7(r)
  Constant10/1 -> Cable Contact Forces/9(mu)
  d_theta/1 -> Newton-Euler Recursive Inverse Dynamics Block/2(d_theta)
  Constant1/1 -> Newton-Euler Recursive Inverse Dynamics Block/4(m)
  Constant5/1 -> Newton-Euler Recursive Inverse Dynamics Block/8(g)
  Newton-Euler Recursive Inverse Dynamics Block/1(u) -> tau/1
  Cable Contact Forces/2(T_ec) -> Newton-Euler Recursive Inverse Dynamics Block/10(T_ec)
  Cable Contact Forces/1(F_ec) -> Newton-Euler Recursive Inverse Dynamics Block/9(F_ec)
  Constant12/1 -> Cable Contact Forces/7(l_link)
  tau_c/1 -> Cable Contact Forces/1(tau_m)

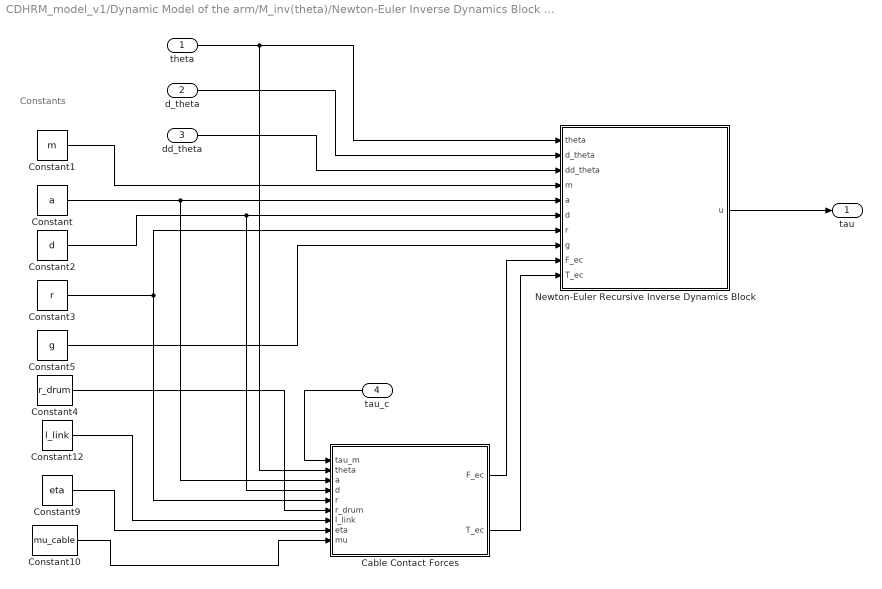
== system CDHRM_model_v1/Dynamic Model of the arm/M_inv(theta)/Newton-Euler Inverse Dynamics Block 14 ==
  note: Constants
  theta : Inport
  d_theta : Inport  Port=2
  dd_theta : Inport  Port=3
  tau_c : Inport  Port=4
  Cable Contact Forces : MATLAB Function  TreatAsAtomicUnit=on
  Constant : Constant  Value=a
  Constant1 : Constant  Value=m
  Constant10 : Constant  Value=mu_cable
  Constant12 : Constant  Value=l_link
  Constant2 : Constant  Value=d
  Constant3 : Constant  Value=r
  Constant4 : Constant  Value=r_drum
  Constant5 : Constant  Value=g
  Constant9 : Constant  Value=eta
  Newton-Euler Recursive Inverse Dynamics Block : MATLAB Function  TreatAsAtomicUnit=on
  tau : Outport
  wires:
  Constant/1 -> Cable Contact Forces/3(a), Newton-Euler Recursive Inverse Dynamics Block/5(a)
  dd_theta/1 -> Newton-Euler Recursive Inverse Dynamics Block/3(dd_theta)
  Constant9/1 -> Cable Contact Forces/8(eta)
  Constant4/1 -> Cable Contact Forces/6(r_drum)
  theta/1 -> Newton-Euler Recursive Inverse Dynamics Block/1(theta), Cable Contact Forces/2(theta)
  Constant2/1 -> Cable Contact Forces/4(d), Newton-Euler Recursive Inverse Dynamics Block/6(d)
  Constant3/1 -> Cable Contact Forces/5(r), Newton-Euler Recursive Inverse Dynamics Block/7(r)
  Constant10/1 -> Cable Contact Forces/9(mu)
  d_theta/1 -> Newton-Euler Recursive Inverse Dynamics Block/2(d_theta)
  Constant1/1 -> Newton-Euler Recursive Inverse Dynamics Block/4(m)
  Constant5/1 -> Newton-Euler Recursive Inverse Dynamics Block/8(g)
  Newton-Euler Recursive Inverse Dynamics Block/1(u) -> tau/1
  Cable Contact Forces/2(T_ec) -> Newton-Euler Recursive Inverse Dynamics Block/10(T_ec)
  Cable Contact Forces/1(F_ec) -> Newton-Euler Recursive Inverse Dynamics Block/9(F_ec)
  Constant12/1 -> Cable Contact Forces/7(l_link)
  tau_c/1 -> Cable Contact Forces/1(tau_m)

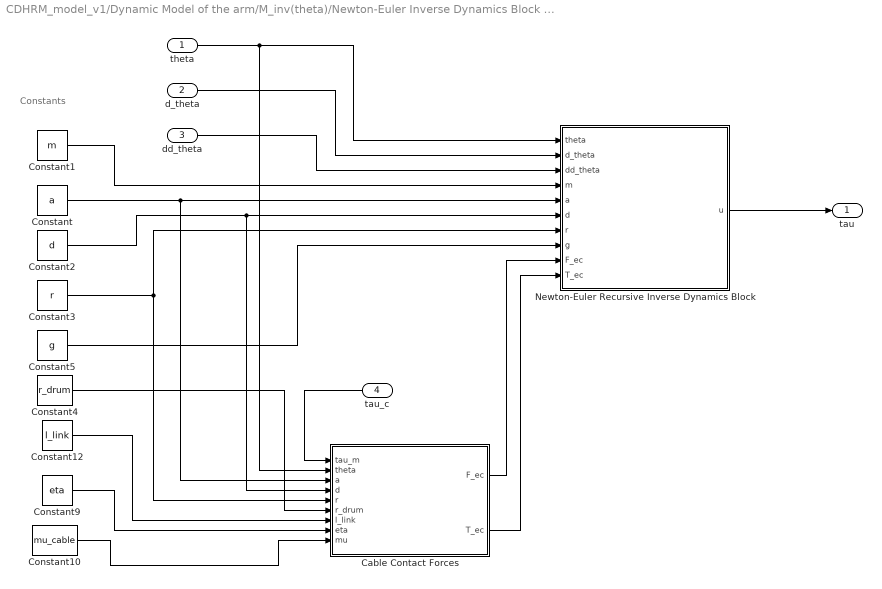
== system CDHRM_model_v1/Dynamic Model of the arm/M_inv(theta)/Newton-Euler Inverse Dynamics Block 15 ==
  note: Constants
  theta : Inport
  d_theta : Inport  Port=2
  dd_theta : Inport  Port=3
  tau_c : Inport  Port=4
  Cable Contact Forces : MATLAB Function  TreatAsAtomicUnit=on
  Constant : Constant  Value=a
  Constant1 : Constant  Value=m
  Constant10 : Constant  Value=mu_cable
  Constant12 : Constant  Value=l_link
  Constant2 : Constant  Value=d
  Constant3 : Constant  Value=r
  Constant4 : Constant  Value=r_drum
  Constant5 : Constant  Value=g
  Constant9 : Constant  Value=eta
  Newton-Euler Recursive Inverse Dynamics Block : MATLAB Function  TreatAsAtomicUnit=on
  tau : Outport
  wires:
  Constant/1 -> Cable Contact Forces/3(a), Newton-Euler Recursive Inverse Dynamics Block/5(a)
  dd_theta/1 -> Newton-Euler Recursive Inverse Dynamics Block/3(dd_theta)
  Constant9/1 -> Cable Contact Forces/8(eta)
  Constant4/1 -> Cable Contact Forces/6(r_drum)
  theta/1 -> Newton-Euler Recursive Inverse Dynamics Block/1(theta), Cable Contact Forces/2(theta)
  Constant2/1 -> Cable Contact Forces/4(d), Newton-Euler Recursive Inverse Dynamics Block/6(d)
  Constant3/1 -> Cable Contact Forces/5(r), Newton-Euler Recursive Inverse Dynamics Block/7(r)
  Constant10/1 -> Cable Contact Forces/9(mu)
  d_theta/1 -> Newton-Euler Recursive Inverse Dynamics Block/2(d_theta)
  Constant1/1 -> Newton-Euler Recursive Inverse Dynamics Block/4(m)
  Constant5/1 -> Newton-Euler Recursive Inverse Dynamics Block/8(g)
  Newton-Euler Recursive Inverse Dynamics Block/1(u) -> tau/1
  Cable Contact Forces/2(T_ec) -> Newton-Euler Recursive Inverse Dynamics Block/10(T_ec)
  Cable Contact Forces/1(F_ec) -> Newton-Euler Recursive Inverse Dynamics Block/9(F_ec)
  Constant12/1 -> Cable Contact Forces/7(l_link)
  tau_c/1 -> Cable Contact Forces/1(tau_m)

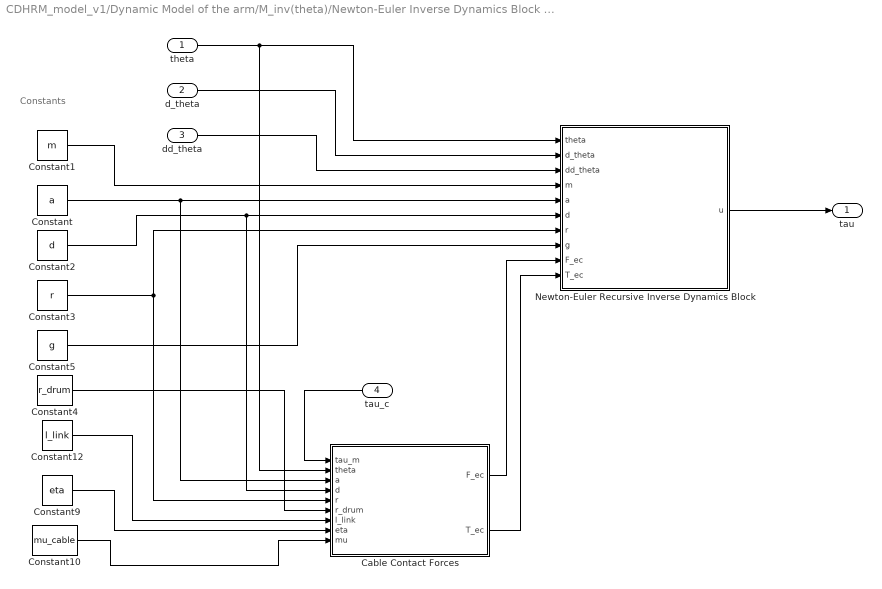
== system CDHRM_model_v1/Dynamic Model of the arm/M_inv(theta)/Newton-Euler Inverse Dynamics Block 16 ==
  note: Constants
  theta : Inport
  d_theta : Inport  Port=2
  dd_theta : Inport  Port=3
  tau_c : Inport  Port=4
  Cable Contact Forces : MATLAB Function  TreatAsAtomicUnit=on
  Constant : Constant  Value=a
  Constant1 : Constant  Value=m
  Constant10 : Constant  Value=mu_cable
  Constant12 : Constant  Value=l_link
  Constant2 : Constant  Value=d
  Constant3 : Constant  Value=r
  Constant4 : Constant  Value=r_drum
  Constant5 : Constant  Value=g
  Constant9 : Constant  Value=eta
  Newton-Euler Recursive Inverse Dynamics Block : MATLAB Function  TreatAsAtomicUnit=on
  tau : Outport
  wires:
  Constant/1 -> Cable Contact Forces/3(a), Newton-Euler Recursive Inverse Dynamics Block/5(a)
  dd_theta/1 -> Newton-Euler Recursive Inverse Dynamics Block/3(dd_theta)
  Constant9/1 -> Cable Contact Forces/8(eta)
  Constant4/1 -> Cable Contact Forces/6(r_drum)
  theta/1 -> Newton-Euler Recursive Inverse Dynamics Block/1(theta), Cable Contact Forces/2(theta)
  Constant2/1 -> Cable Contact Forces/4(d), Newton-Euler Recursive Inverse Dynamics Block/6(d)
  Constant3/1 -> Cable Contact Forces/5(r), Newton-Euler Recursive Inverse Dynamics Block/7(r)
  Constant10/1 -> Cable Contact Forces/9(mu)
  d_theta/1 -> Newton-Euler Recursive Inverse Dynamics Block/2(d_theta)
  Constant1/1 -> Newton-Euler Recursive Inverse Dynamics Block/4(m)
  Constant5/1 -> Newton-Euler Recursive Inverse Dynamics Block/8(g)
  Newton-Euler Recursive Inverse Dynamics Block/1(u) -> tau/1
  Cable Contact Forces/2(T_ec) -> Newton-Euler Recursive Inverse Dynamics Block/10(T_ec)
  Cable Contact Forces/1(F_ec) -> Newton-Euler Recursive Inverse Dynamics Block/9(F_ec)
  Constant12/1 -> Cable Contact Forces/7(l_link)
  tau_c/1 -> Cable Contact Forces/1(tau_m)

== system CDHRM_model_v1/Dynamic Model of the arm/M_inv(theta)/Newton-Euler Inverse Dynamics Block 17 ==
  note: Constants
  theta : Inport
  d_theta : Inport  Port=2
  dd_theta : Inport  Port=3
  tau_c : Inport  Port=4
  Cable Contact Forces : MATLAB Function  TreatAsAtomicUnit=on
  Constant : Constant  Value=a
  Constant1 : Constant  Value=m
  Constant10 : Constant  Value=mu_cable
  Constant12 : Constant  Value=l_link
  Constant2 : Constant  Value=d
  Constant3 : Constant  Value=r
  Constant4 : Constant  Value=r_drum
  Constant5 : Constant  Value=g
  Constant9 : Constant  Value=eta
  Newton-Euler Recursive Inverse Dynamics Block : MATLAB Function  TreatAsAtomicUnit=on
  tau : Outport
  wires:
  Constant/1 -> Cable Contact Forces/3(a), Newton-Euler Recursive Inverse Dynamics Block/5(a)
  dd_theta/1 -> Newton-Euler Recursive Inverse Dynamics Block/3(dd_theta)
  Constant9/1 -> Cable Contact Forces/8(eta)
  Constant4/1 -> Cable Contact Forces/6(r_drum)
  theta/1 -> Newton-Euler Recursive Inverse Dynamics Block/1(theta), Cable Contact Forces/2(theta)
  Constant2/1 -> Cable Contact Forces/4(d), Newton-Euler Recursive Inverse Dynamics Block/6(d)
  Constant3/1 -> Cable Contact Forces/5(r), Newton-Euler Recursive Inverse Dynamics Block/7(r)
  Constant10/1 -> Cable Contact Forces/9(mu)
  d_theta/1 -> Newton-Euler Recursive Inverse Dynamics Block/2(d_theta)
  Constant1/1 -> Newton-Euler Recursive Inverse Dynamics Block/4(m)
  Constant5/1 -> Newton-Euler Recursive Inverse Dynamics Block/8(g)
  Newton-Euler Recursive Inverse Dynamics Block/1(u) -> tau/1
  Cable Contact Forces/2(T_ec) -> Newton-Euler Recursive Inverse Dynamics Block/10(T_ec)
  Cable Contact Forces/1(F_ec) -> Newton-Euler Recursive Inverse Dynamics Block/9(F_ec)
  Constant12/1 -> Cable Contact Forces/7(l_link)
  tau_c/1 -> Cable Contact Forces/1(tau_m)

== system CDHRM_model_v1/Dynamic Model of the arm/M_inv(theta)/Newton-Euler Inverse Dynamics Block 2 ==
  note: Constants
  theta : Inport
  d_theta : Inport  Port=2
  dd_theta : Inport  Port=3
  tau_c : Inport  Port=4
  Cable Contact Forces : MATLAB Function  TreatAsAtomicUnit=on
  Constant : Constant  Value=a
  Constant1 : Constant  Value=m
  Constant10 : Constant  Value=mu_cable
  Constant12 : Constant  Value=l_link
  Constant2 : Constant  Value=d
  Constant3 : Constant  Value=r
  Constant4 : Constant  Value=r_drum
  Constant5 : Constant  Value=g
  Constant9 : Constant  Value=eta
  Newton-Euler Recursive Inverse Dynamics Block : MATLAB Function  TreatAsAtomicUnit=on
  tau : Outport
  wires:
  Constant/1 -> Cable Contact Forces/3(a), Newton-Euler Recursive Inverse Dynamics Block/5(a)
  dd_theta/1 -> Newton-Euler Recursive Inverse Dynamics Block/3(dd_theta)
  Constant9/1 -> Cable Contact Forces/8(eta)
  Constant4/1 -> Cable Contact Forces/6(r_drum)
  theta/1 -> Newton-Euler Recursive Inverse Dynamics Block/1(theta), Cable Contact Forces/2(theta)
  Constant2/1 -> Cable Contact Forces/4(d), Newton-Euler Recursive Inverse Dynamics Block/6(d)
  Constant3/1 -> Cable Contact Forces/5(r), Newton-Euler Recursive Inverse Dynamics Block/7(r)
  Constant10/1 -> Cable Contact Forces/9(mu)
  d_theta/1 -> Newton-Euler Recursive Inverse Dynamics Block/2(d_theta)
  Constant1/1 -> Newton-Euler Recursive Inverse Dynamics Block/4(m)
  Constant5/1 -> Newton-Euler Recursive Inverse Dynamics Block/8(g)
  Newton-Euler Recursive Inverse Dynamics Block/1(u) -> tau/1
  Cable Contact Forces/2(T_ec) -> Newton-Euler Recursive Inverse Dynamics Block/10(T_ec)
  Cable Contact Forces/1(F_ec) -> Newton-Euler Recursive Inverse Dynamics Block/9(F_ec)
  Constant12/1 -> Cable Contact Forces/7(l_link)
  tau_c/1 -> Cable Contact Forces/1(tau_m)

== system CDHRM_model_v1/Dynamic Model of the arm/M_inv(theta)/Newton-Euler Inverse Dynamics Block 3 ==
  note: Constants
  theta : Inport
  d_theta : Inport  Port=2
  dd_theta : Inport  Port=3
  tau_c : Inport  Port=4
  Cable Contact Forces : MATLAB Function  TreatAsAtomicUnit=on
  Constant : Constant  Value=a
  Constant1 : Constant  Value=m
  Constant10 : Constant  Value=mu_cable
  Constant12 : Constant  Value=l_link
  Constant2 : Constant  Value=d
  Constant3 : Constant  Value=r
  Constant4 : Constant  Value=r_drum
  Constant5 : Constant  Value=g
  Constant9 : Constant  Value=eta
  Newton-Euler Recursive Inverse Dynamics Block : MATLAB Function  TreatAsAtomicUnit=on
  tau : Outport
  wires:
  Constant/1 -> Cable Contact Forces/3(a), Newton-Euler Recursive Inverse Dynamics Block/5(a)
  dd_theta/1 -> Newton-Euler Recursive Inverse Dynamics Block/3(dd_theta)
  Constant9/1 -> Cable Contact Forces/8(eta)
  Constant4/1 -> Cable Contact Forces/6(r_drum)
  theta/1 -> Newton-Euler Recursive Inverse Dynamics Block/1(theta), Cable Contact Forces/2(theta)
  Constant2/1 -> Cable Contact Forces/4(d), Newton-Euler Recursive Inverse Dynamics Block/6(d)
  Constant3/1 -> Cable Contact Forces/5(r), Newton-Euler Recursive Inverse Dynamics Block/7(r)
  Constant10/1 -> Cable Contact Forces/9(mu)
  d_theta/1 -> Newton-Euler Recursive Inverse Dynamics Block/2(d_theta)
  Constant1/1 -> Newton-Euler Recursive Inverse Dynamics Block/4(m)
  Constant5/1 -> Newton-Euler Recursive Inverse Dynamics Block/8(g)
  Newton-Euler Recursive Inverse Dynamics Block/1(u) -> tau/1
  Cable Contact Forces/2(T_ec) -> Newton-Euler Recursive Inverse Dynamics Block/10(T_ec)
  Cable Contact Forces/1(F_ec) -> Newton-Euler Recursive Inverse Dynamics Block/9(F_ec)
  Constant12/1 -> Cable Contact Forces/7(l_link)
  tau_c/1 -> Cable Contact Forces/1(tau_m)

== system CDHRM_model_v1/Dynamic Model of the arm/M_inv(theta)/Newton-Euler Inverse Dynamics Block 4 ==
  note: Constants
  theta : Inport
  d_theta : Inport  Port=2
  dd_theta : Inport  Port=3
  tau_c : Inport  Port=4
  Cable Contact Forces : MATLAB Function  TreatAsAtomicUnit=on
  Constant : Constant  Value=a
  Constant1 : Constant  Value=m
  Constant10 : Constant  Value=mu_cable
  Constant12 : Constant  Value=l_link
  Constant2 : Constant  Value=d
  Constant3 : Constant  Value=r
  Constant4 : Constant  Value=r_drum
  Constant5 : Constant  Value=g
  Constant9 : Constant  Value=eta
  Newton-Euler Recursive Inverse Dynamics Block : MATLAB Function  TreatAsAtomicUnit=on
  tau : Outport
  wires:
  Constant/1 -> Cable Contact Forces/3(a), Newton-Euler Recursive Inverse Dynamics Block/5(a)
  dd_theta/1 -> Newton-Euler Recursive Inverse Dynamics Block/3(dd_theta)
  Constant9/1 -> Cable Contact Forces/8(eta)
  Constant4/1 -> Cable Contact Forces/6(r_drum)
  theta/1 -> Newton-Euler Recursive Inverse Dynamics Block/1(theta), Cable Contact Forces/2(theta)
  Constant2/1 -> Cable Contact Forces/4(d), Newton-Euler Recursive Inverse Dynamics Block/6(d)
  Constant3/1 -> Cable Contact Forces/5(r), Newton-Euler Recursive Inverse Dynamics Block/7(r)
  Constant10/1 -> Cable Contact Forces/9(mu)
  d_theta/1 -> Newton-Euler Recursive Inverse Dynamics Block/2(d_theta)
  Constant1/1 -> Newton-Euler Recursive Inverse Dynamics Block/4(m)
  Constant5/1 -> Newton-Euler Recursive Inverse Dynamics Block/8(g)
  Newton-Euler Recursive Inverse Dynamics Block/1(u) -> tau/1
  Cable Contact Forces/2(T_ec) -> Newton-Euler Recursive Inverse Dynamics Block/10(T_ec)
  Cable Contact Forces/1(F_ec) -> Newton-Euler Recursive Inverse Dynamics Block/9(F_ec)
  Constant12/1 -> Cable Contact Forces/7(l_link)
  tau_c/1 -> Cable Contact Forces/1(tau_m)

== system CDHRM_model_v1/Dynamic Model of the arm/M_inv(theta)/Newton-Euler Inverse Dynamics Block 5 ==
  note: Constants
  theta : Inport
  d_theta : Inport  Port=2
  dd_theta : Inport  Port=3
  tau_c : Inport  Port=4
  Cable Contact Forces : MATLAB Function  TreatAsAtomicUnit=on
  Constant : Constant  Value=a
  Constant1 : Constant  Value=m
  Constant10 : Constant  Value=mu_cable
  Constant12 : Constant  Value=l_link
  Constant2 : Constant  Value=d
  Constant3 : Constant  Value=r
  Constant4 : Constant  Value=r_drum
  Constant5 : Constant  Value=g
  Constant9 : Constant  Value=eta
  Newton-Euler Recursive Inverse Dynamics Block : MATLAB Function  TreatAsAtomicUnit=on
  tau : Outport
  wires:
  Constant/1 -> Cable Contact Forces/3(a), Newton-Euler Recursive Inverse Dynamics Block/5(a)
  dd_theta/1 -> Newton-Euler Recursive Inverse Dynamics Block/3(dd_theta)
  Constant9/1 -> Cable Contact Forces/8(eta)
  Constant4/1 -> Cable Contact Forces/6(r_drum)
  theta/1 -> Newton-Euler Recursive Inverse Dynamics Block/1(theta), Cable Contact Forces/2(theta)
  Constant2/1 -> Cable Contact Forces/4(d), Newton-Euler Recursive Inverse Dynamics Block/6(d)
  Constant3/1 -> Cable Contact Forces/5(r), Newton-Euler Recursive Inverse Dynamics Block/7(r)
  Constant10/1 -> Cable Contact Forces/9(mu)
  d_theta/1 -> Newton-Euler Recursive Inverse Dynamics Block/2(d_theta)
  Constant1/1 -> Newton-Euler Recursive Inverse Dynamics Block/4(m)
  Constant5/1 -> Newton-Euler Recursive Inverse Dynamics Block/8(g)
  Newton-Euler Recursive Inverse Dynamics Block/1(u) -> tau/1
  Cable Contact Forces/2(T_ec) -> Newton-Euler Recursive Inverse Dynamics Block/10(T_ec)
  Cable Contact Forces/1(F_ec) -> Newton-Euler Recursive Inverse Dynamics Block/9(F_ec)
  Constant12/1 -> Cable Contact Forces/7(l_link)
  tau_c/1 -> Cable Contact Forces/1(tau_m)

== system CDHRM_model_v1/Dynamic Model of the arm/M_inv(theta)/Newton-Euler Inverse Dynamics Block 6 ==
  note: Constants
  theta : Inport
  d_theta : Inport  Port=2
  dd_theta : Inport  Port=3
  tau_c : Inport  Port=4
  Cable Contact Forces : MATLAB Function  TreatAsAtomicUnit=on
  Constant : Constant  Value=a
  Constant1 : Constant  Value=m
  Constant10 : Constant  Value=mu_cable
  Constant12 : Constant  Value=l_link
  Constant2 : Constant  Value=d
  Constant3 : Constant  Value=r
  Constant4 : Constant  Value=r_drum
  Constant5 : Constant  Value=g
  Constant9 : Constant  Value=eta
  Newton-Euler Recursive Inverse Dynamics Block : MATLAB Function  TreatAsAtomicUnit=on
  tau : Outport
  wires:
  Constant/1 -> Cable Contact Forces/3(a), Newton-Euler Recursive Inverse Dynamics Block/5(a)
  dd_theta/1 -> Newton-Euler Recursive Inverse Dynamics Block/3(dd_theta)
  Constant9/1 -> Cable Contact Forces/8(eta)
  Constant4/1 -> Cable Contact Forces/6(r_drum)
  theta/1 -> Newton-Euler Recursive Inverse Dynamics Block/1(theta), Cable Contact Forces/2(theta)
  Constant2/1 -> Cable Contact Forces/4(d), Newton-Euler Recursive Inverse Dynamics Block/6(d)
  Constant3/1 -> Cable Contact Forces/5(r), Newton-Euler Recursive Inverse Dynamics Block/7(r)
  Constant10/1 -> Cable Contact Forces/9(mu)
  d_theta/1 -> Newton-Euler Recursive Inverse Dynamics Block/2(d_theta)
  Constant1/1 -> Newton-Euler Recursive Inverse Dynamics Block/4(m)
  Constant5/1 -> Newton-Euler Recursive Inverse Dynamics Block/8(g)
  Newton-Euler Recursive Inverse Dynamics Block/1(u) -> tau/1
  Cable Contact Forces/2(T_ec) -> Newton-Euler Recursive Inverse Dynamics Block/10(T_ec)
  Cable Contact Forces/1(F_ec) -> Newton-Euler Recursive Inverse Dynamics Block/9(F_ec)
  Constant12/1 -> Cable Contact Forces/7(l_link)
  tau_c/1 -> Cable Contact Forces/1(tau_m)

== system CDHRM_model_v1/Dynamic Model of the arm/M_inv(theta)/Newton-Euler Inverse Dynamics Block 7 ==
  note: Constants
  theta : Inport
  d_theta : Inport  Port=2
  dd_theta : Inport  Port=3
  tau_c : Inport  Port=4
  Cable Contact Forces : MATLAB Function  TreatAsAtomicUnit=on
  Constant : Constant  Value=a
  Constant1 : Constant  Value=m
  Constant10 : Constant  Value=mu_cable
  Constant12 : Constant  Value=l_link
  Constant2 : Constant  Value=d
  Constant3 : Constant  Value=r
  Constant4 : Constant  Value=r_drum
  Constant5 : Constant  Value=g
  Constant9 : Constant  Value=eta
  Newton-Euler Recursive Inverse Dynamics Block : MATLAB Function  TreatAsAtomicUnit=on
  tau : Outport
  wires:
  Constant/1 -> Cable Contact Forces/3(a), Newton-Euler Recursive Inverse Dynamics Block/5(a)
  dd_theta/1 -> Newton-Euler Recursive Inverse Dynamics Block/3(dd_theta)
  Constant9/1 -> Cable Contact Forces/8(eta)
  Constant4/1 -> Cable Contact Forces/6(r_drum)
  theta/1 -> Newton-Euler Recursive Inverse Dynamics Block/1(theta), Cable Contact Forces/2(theta)
  Constant2/1 -> Cable Contact Forces/4(d), Newton-Euler Recursive Inverse Dynamics Block/6(d)
  Constant3/1 -> Cable Contact Forces/5(r), Newton-Euler Recursive Inverse Dynamics Block/7(r)
  Constant10/1 -> Cable Contact Forces/9(mu)
  d_theta/1 -> Newton-Euler Recursive Inverse Dynamics Block/2(d_theta)
  Constant1/1 -> Newton-Euler Recursive Inverse Dynamics Block/4(m)
  Constant5/1 -> Newton-Euler Recursive Inverse Dynamics Block/8(g)
  Newton-Euler Recursive Inverse Dynamics Block/1(u) -> tau/1
  Cable Contact Forces/2(T_ec) -> Newton-Euler Recursive Inverse Dynamics Block/10(T_ec)
  Cable Contact Forces/1(F_ec) -> Newton-Euler Recursive Inverse Dynamics Block/9(F_ec)
  Constant12/1 -> Cable Contact Forces/7(l_link)
  tau_c/1 -> Cable Contact Forces/1(tau_m)
